simulink model "battery_pack_100s2p"  (R2025b)
settings: Solver=daessc  StartTime=0.0  StopTime=5970.0  MaxStep=5  RelTol=1e-3  AbsTol=1e-4
PostLoadFcn:
  | addpath(fullfile(fileparts(which(bdroot)),'generated'));
model workspace (MAT data in the model file):
  IpackTS = timeseries
  IpackTS.Name = 'unnamed'
  IpackTS.DataInfo = tsdata.datametadata
  IpackTS.DataInfo.Interpolation = tsdata.interpolation
  IpackTS.DataInfo.Interpolation.Fhandle : function handle (value not decoded)
  IpackTS.DataInfo.Interpolation.Name = 'linear'
  IpackTS.TimeInfo = tsdata.timemetadata
  IpackTS.TimeInfo.Length = 10
  IpackTS.TimeInfo.DuplicateTimes = 0
  IpackTS.TimeInfo.Time_ = [0; 60; 61; 2940; 2941; 3540; 3541; 5070; 5071; 5970]
  IpackTS.TimeInfo.Initialized = 1
  IpackTS.QualityInfo = tsdata.qualmetadata
  IpackTS.Data_ = [0; 0; -9; -9; 0; 0; 18; 18; 0; 0]
  ModuleBot.SOC_vecCell = [0 0.05 0.1 0.2 0.3 0.4 0.5 0.6 0.7 0.8 0.9 0.95 1]
  ModuleBot.T_vecCell = [273.15 298.15 323.15]
  ModuleBot.V0_matCell = [2.99  3  3.006; 3.34  3.35  3.356; 3.44  3.45  3.456; 3.54  3.55  3.556; 3.61  3.62  3.626; 3.67  3.68  3.686; 3.74  3.75  3.756; 3.82  3.83  3.836; 3.92  3.93  3.936; 4.01  4.02  4.026; 4.11  4.12  4.126; 4.16  4.17  4.176; 4.19  4.2  4.206]
  ModuleBot.V_rangeCell = [0 Inf]
  ModuleBot.R0_matCell = [0.0386100001983  0.0297000001525  0.0207900001068; 0.0339579673557  0.0261215133506  0.0182850593454; 0.0314679140664  0.0242060877434  0.0169442614204; 0.0294216763947  0.0226320587651  0.0158424411356; 0.0288354420652  0.0221811092809  0.0155267764967; 0.028667602662  0.0220520020477  0.0154364014334; 0.0286201487939  0.0220154990723  0.0154108493506; 0.0286099040538  0.0220076185029  0.015405332952; 0.028624710832  0.0220190083323  0.0154133058326; 0.0287228875985  0.0220945289219  0.0154661702453; 0.029248351272  0.0224987317477  0.0157491122234; 0.0300916107443  0.0231473928802  0.0162031750161; 0.0320320373038  0.0246400286952  0.0172480200867]
  ModuleBot.AHCell = 4.5
  ModuleBot.thermal_massCell = 63
  ModuleBot.AmbientResistance = 34
  ModuleBot.XminThermalResistance = 25
  ModuleBot.InterCellThermalResistance = 50
  ModuleBot.InterParallelAssemblyThermalResistance = [50 142.857142857 142.857142857 50 50 142.857142857 142.857142857 50 50 142.857142857 142.857142857 50 50 142.857142857 142.857142857 50 50 142.857142857 142.857142857 50 50 142.857142857 142.857142857 50 50 142.857142857 142.857142857 50 50 142.857142857 142.857142857 50 50 142.857142857 142.857142857 50]
  ModuleBot.InterCellRadiationArea = 0.00045
  ModuleBot.InterCellRadiationCoefficient = 4.8198179e-08
  ModuleBot.InterParallelAssemblyRadiationArea = [0.00045 0.00012 0.00012 0.00045 0.00045 0.00012 0.00012 0.00045 0.00045 0.00012 0.00012 0.00045 0.00045 0.00012 0.00012 0.00045 0.00045 0.00012 0.00012 0.00045 0.00045 0.00012 0.00012 0.00045 0.00045 0.00012 0.00012 0.00045 0.00045 0.00012 0.00012 0.00045 0.00045 0.00012 0.00012 0.00045]
  ModuleBot.InterParallelAssemblyRadiationCoefficient = 4.8198179e-08
  ModuleMid.SOC_vecCell = [0 0.05 0.1 0.2 0.3 0.4 0.5 0.6 0.7 0.8 0.9 0.95 1]
  ModuleMid.T_vecCell = [273.15 298.15 323.15]
  ModuleMid.V0_matCell = [2.99  3  3.006; 3.34  3.35  3.356; 3.44  3.45  3.456; 3.54  3.55  3.556; 3.61  3.62  3.626; 3.67  3.68  3.686; 3.74  3.75  3.756; 3.82  3.83  3.836; 3.92  3.93  3.936; 4.01  4.02  4.026; 4.11  4.12  4.126; 4.16  4.17  4.176; 4.19  4.2  4.206]
  ModuleMid.V_rangeCell = [0 Inf]
  ModuleMid.R0_matCell = [0.0386100001983  0.0297000001525  0.0207900001068; 0.0339579673557  0.0261215133506  0.0182850593454; 0.0314679140664  0.0242060877434  0.0169442614204; 0.0294216763947  0.0226320587651  0.0158424411356; 0.0288354420652  0.0221811092809  0.0155267764967; 0.028667602662  0.0220520020477  0.0154364014334; 0.0286201487939  0.0220154990723  0.0154108493506; 0.0286099040538  0.0220076185029  0.015405332952; 0.028624710832  0.0220190083323  0.0154133058326; 0.0287228875985  0.0220945289219  0.0154661702453; 0.029248351272  0.0224987317477  0.0157491122234; 0.0300916107443  0.0231473928802  0.0162031750161; 0.0320320373038  0.0246400286952  0.0172480200867]
  ModuleMid.AHCell = 4.5
  ModuleMid.thermal_massCell = 63
  ModuleMid.AmbientResistance = 34
  ModuleMid.XminThermalResistance = 25
  ModuleMid.XmaxThermalResistance = 25
  ModuleMid.InterCellThermalResistance = 50
  ModuleMid.InterParallelAssemblyThermalResistance = [50 142.857142857 142.857142857 50 50 142.857142857 142.857142857 50 50 142.857142857 142.857142857 50 50 142.857142857 142.857142857 50 50 142.857142857 142.857142857 50 50 142.857142857 142.857142857 50 50 142.857142857 142.857142857 50 50 142.857142857 142.857142857 50 50 142.857142857 142.857142857 50]
  ModuleMid.InterCellRadiationArea = 0.00045
  ModuleMid.InterCellRadiationCoefficient = 4.8198179e-08
  ModuleMid.InterParallelAssemblyRadiationArea = [0.00045 0.00012 0.00012 0.00045 0.00045 0.00012 0.00012 0.00045 0.00045 0.00012 0.00012 0.00045 0.00045 0.00012 0.00012 0.00045 0.00045 0.00012 0.00012 0.00045 0.00045 0.00012 0.00012 0.00045 0.00045 0.00012 0.00012 0.00045 0.00045 0.00012 0.00012 0.00045 0.00045 0.00012 0.00012 0.00045]
  ModuleMid.InterParallelAssemblyRadiationCoefficient = 4.8198179e-08
  ModuleTop.SOC_vecCell = [0 0.05 0.1 0.2 0.3 0.4 0.5 0.6 0.7 0.8 0.9 0.95 1]
  ModuleTop.T_vecCell = [273.15 298.15 323.15]
  ModuleTop.V0_matCell = [2.99  3  3.006; 3.34  3.35  3.356; 3.44  3.45  3.456; 3.54  3.55  3.556; 3.61  3.62  3.626; 3.67  3.68  3.686; 3.74  3.75  3.756; 3.82  3.83  3.836; 3.92  3.93  3.936; 4.01  4.02  4.026; 4.11  4.12  4.126; 4.16  4.17  4.176; 4.19  4.2  4.206]
  ModuleTop.V_rangeCell = [0 Inf]
  ModuleTop.R0_matCell = [0.0386100001983  0.0297000001525  0.0207900001068; 0.0339579673557  0.0261215133506  0.0182850593454; 0.0314679140664  0.0242060877434  0.0169442614204; 0.0294216763947  0.0226320587651  0.0158424411356; 0.0288354420652  0.0221811092809  0.0155267764967; 0.028667602662  0.0220520020477  0.0154364014334; 0.0286201487939  0.0220154990723  0.0154108493506; 0.0286099040538  0.0220076185029  0.015405332952; 0.028624710832  0.0220190083323  0.0154133058326; 0.0287228875985  0.0220945289219  0.0154661702453; 0.029248351272  0.0224987317477  0.0157491122234; 0.0300916107443  0.0231473928802  0.0162031750161; 0.0320320373038  0.0246400286952  0.0172480200867]
  ModuleTop.AHCell = 4.5
  ModuleTop.thermal_massCell = 63
  ModuleTop.AmbientResistance = 34
  ModuleTop.XmaxThermalResistance = 25
  ModuleTop.InterCellThermalResistance = 50
  ModuleTop.InterParallelAssemblyThermalResistance = [50 142.857142857 142.857142857 50 50 142.857142857 142.857142857 50 50 142.857142857 142.857142857 50 50 142.857142857 142.857142857 50 50 142.857142857 142.857142857 50 50 142.857142857 142.857142857 50 50 142.857142857 142.857142857 50 50 142.857142857 142.857142857 50 50 142.857142857 142.857142857 50]
  ModuleTop.InterCellRadiationArea = 0.00045
  ModuleTop.InterCellRadiationCoefficient = 4.8198179e-08
  ModuleTop.InterParallelAssemblyRadiationArea = [0.00045 0.00012 0.00012 0.00045 0.00045 0.00012 0.00012 0.00045 0.00045 0.00012 0.00012 0.00045 0.00045 0.00012 0.00012 0.00045 0.00045 0.00012 0.00012 0.00045 0.00045 0.00012 0.00012 0.00045 0.00045 0.00012 0.00012 0.00045 0.00045 0.00012 0.00012 0.00045 0.00045 0.00012 0.00012 0.00045]
  ModuleTop.InterParallelAssemblyRadiationCoefficient = 4.8198179e-08
  ParallelAssemblyType1.SOC_vecCell = [0 0.05 0.1 0.2 0.3 0.4 0.5 0.6 0.7 0.8 0.9 0.95 1]
  ParallelAssemblyType1.T_vecCell = [273.15 298.15 323.15]
  ParallelAssemblyType1.V0_matCell = [2.99  3  3.006; 3.34  3.35  3.356; 3.44  3.45  3.456; 3.54  3.55  3.556; 3.61  3.62  3.626; 3.67  3.68  3.686; 3.74  3.75  3.756; 3.82  3.83  3.836; 3.92  3.93  3.936; 4.01  4.02  4.026; 4.11  4.12  4.126; 4.16  4.17  4.176; 4.19  4.2  4.206]
  ParallelAssemblyType1.V_rangeCell = [0 Inf]
  ParallelAssemblyType1.R0_matCell = [0.0386100001983  0.0297000001525  0.0207900001068; 0.0339579673557  0.0261215133506  0.0182850593454; 0.0314679140664  0.0242060877434  0.0169442614204; 0.0294216763947  0.0226320587651  0.0158424411356; 0.0288354420652  0.0221811092809  0.0155267764967; 0.028667602662  0.0220520020477  0.0154364014334; 0.0286201487939  0.0220154990723  0.0154108493506; 0.0286099040538  0.0220076185029  0.015405332952; 0.028624710832  0.0220190083323  0.0154133058326; 0.0287228875985  0.0220945289219  0.0154661702453; 0.029248351272  0.0224987317477  0.0157491122234; 0.0300916107443  0.0231473928802  0.0162031750161; 0.0320320373038  0.0246400286952  0.0172480200867]
  ParallelAssemblyType1.AHCell = 4.5
  ParallelAssemblyType1.thermal_massCell = 63
  ParallelAssemblyType1.AmbientResistance = 34
  ParallelAssemblyType1.XminThermalResistance = 25
  ParallelAssemblyType1.InterCellThermalResistance = 50
  ParallelAssemblyType1.InterCellRadiationArea = 0.00045
  ParallelAssemblyType1.InterCellRadiationCoefficient = 4.8198179e-08
libraries: batt21700_mid_lib x8, fl_lib x4, nesl_utility x3, batt21700_top_lib x1, batt21700_bot_lib x1
settings Model: Creator=nhamb  LastModifiedBy=nhamb
settings SimscapeCC: SimscapeLogType=all

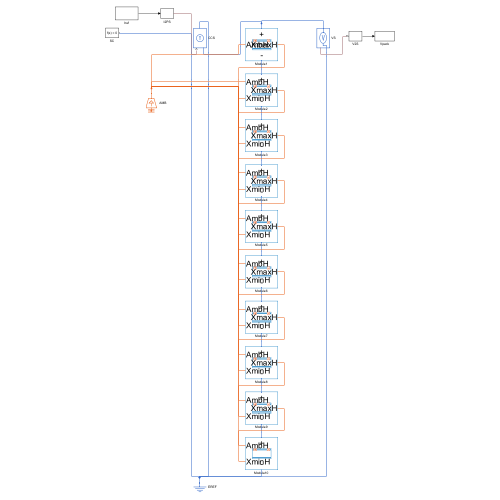
[thumbnail: Simulink's stored preview of the top-level diagram]
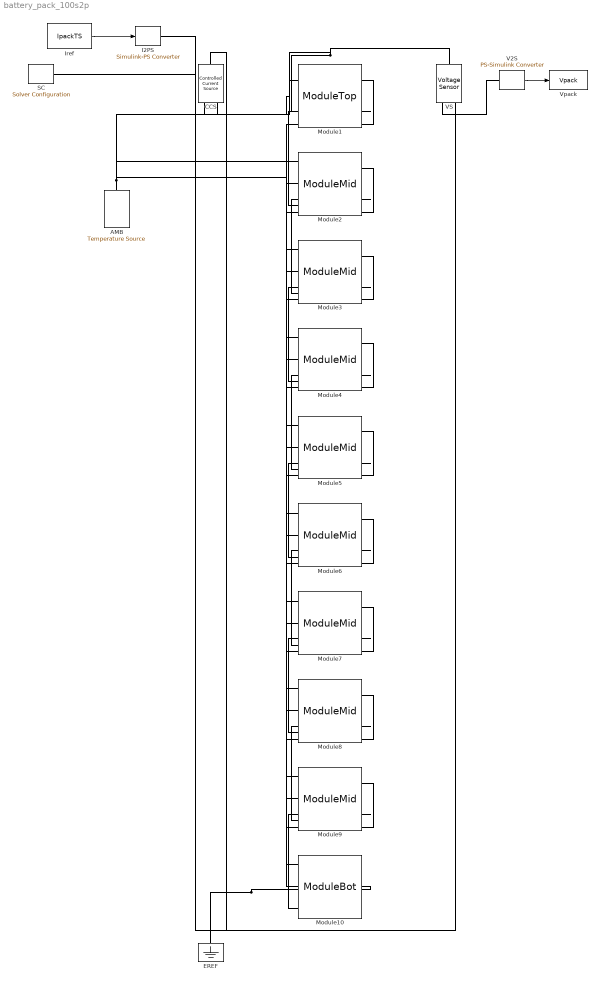
== system battery_pack_100s2p ==
  AMB : fl_lib/Thermal/Thermal Sources/Temperature Source  temperature=298.1500 K
  CCS : fl_lib/Electrical/Electrical Sources/Controlled Current Source
  EREF : fl_lib/Electrical/Electrical Elements/Electrical Reference
  I2PS : nesl_utility/Simulink-PS Converter  PhysicalDomain=network_engine_domain  SubClassName=ps_input  LeftPortType=input  RightPortType=output  PseudoPeriodic=off  Frequencies=[]  NoiseDistribution=none  NoiseParameters=[]  Unit=A  AffineConversion=off  FilteringAndDerivatives=provide  SimscapeFilterOrder=1  InputFilterTimeConstant=0.001  UdotUserProvided=0
  Iref : FromWorkspace  VariableName=IpackTS  OutputAfterFinalValue=Holding final value
  Module1 : batt21700_top_lib/ModuleTop  SOC_vecCell=ModuleTop.SOC_vecCell  T_vecCell=ModuleTop.T_vecCell K  V0_matCell=ModuleTop.V0_matCell V  V_rangeCell=ModuleTop.V_rangeCell V  R0_matCell=ModuleTop.R0_matCell Ohm  AHCell=ModuleTop.AHCell A*hr  extrapolation_optionCell=simscape.enum.extrapolation.nearest  thermal_massCell=ModuleTop.thermal_massCell J/K  AmbientResistance=[22.2034 26.9369 26.9369 34.2356 26.9369 34.2356 26.9369 34.2356 26.9369 34.2356 26.9369 34.2356 26.9369 34.2356 26.9369 34.2356 26.9369 34.2356 22.2034 26.9369] K/W  XmaxThermalResistance=ModuleTop.XmaxThermalResistance K/W  InterCellThermalResistance=ModuleTop.InterCellThermalResistance K/W  InterParallelAssemblyThermalResistance=ModuleTop.InterParallelAssemblyThermalResistance K/W  InterCellRadiationArea=ModuleTop.InterCellRadiationArea m^2  InterCellRadiationCoefficient=ModuleTop.InterCellRadiationCoefficient W/(K^4*m^2)  InterParallelAssemblyRadiationArea=ModuleTop.InterParallelAssemblyRadiationArea m^2  InterParallelAssemblyRadiationCoefficient=ModuleTop.InterParallelAssemblyRadiationCoefficient W/(K^4*m^2)  P=2  S=10  NumInterCellThermalConnections=10  NumInterParallelAssemblyThermalConnections=36  InterParallelAssemblyConnectionsMapping=[1, 1, 1, 1, 2, 2, 2, 2, 3, 3, 3, 3, 4, 4, 4, 4, 5, 5, 5, 5, 6, 6, 6, 6, 7, 7, 7, 7, 8, 8, 8, 8, 9, 9, 9, 9; 2, 2, 2, 2, 3, 3, 3, 3, 4, 4, 4, 4, 5, 5, 5, 5, 6, 6, 6, 6, 7, 7, 7, 7, 8, 8, 8, 8, 9, 9, 9, 9, 10, 10, 10, 10]  InterParallelAssemblyCellConnectionsMapping=[1, 1, 2, 2, 1, 1, 2, 2, 1, 1, 2, 2, 1, 1, 2, 2, 1, 1, 2, 2, 1, 1, 2, 2, 1, 1, 2, 2, 1, 1, 2, 2, 1, 1, 2, 2; 1, 2, 1, 2, 1, 2, 1, 2, 1, 2, 1, 2, 1, 2, 1, 2, 1, 2, 1, 2, 1, 2, 1, 2, 1, 2, 1, 2, 1, 2, 1, 2, 1, 2, 1, 2]  InterCellConnectionsMapping=[1, 1, 1, 1, 1, 1, 1, 1, 1, 1; 2, 2, 2, 2, 2, 2, 2, 2, 2, 2]  NumXmaxConnections=10  XmaxConnectionsMapping=[2, 4, 6, 8, 10, 12, 14, 16, 18, 20]  NumCellsAtXmaxBoundary=10  CellsInModelAtXmaxBoundary=[1, 1, 1, 1, 1, 1, 1, 1, 1, 1]  iCell_specify=off  iCell_priority=None  iCell=repmat(0, 20, 1) A  iCell_nominal_specify=off  iCell_nominal_value=1  iCell_nominal_unit=A  vCell_specify=off  vCell_priority=None  vCell=repmat(0, 20, 1) V  vCell_nominal_specify=off  vCell_nominal_value=1  vCell_nominal_unit=V  socCell_specify=on  socCell_priority=High  socCell=repmat(0.1500,20,1)  socCell_nominal_specify=off  socCell_nominal_value=1  socCell_nominal_unit=1  numCyclesCell_specify=off  numCyclesCell_priority=High  numCyclesCell=repmat(0, 20, 1)  numCyclesCell_nominal_specify=off  numCyclesCell_nominal_value=1  numCyclesCell_nominal_unit=1  temperatureCell_specify=on  temperatureCell_priority=High  temperatureCell=repmat(298.1500,20,1) K  temperatureCell_nominal_specify=off  temperatureCell_nominal_value=1  temperatureCell_nominal_unit=K  vParallelAssembly_specify=off  vParallelAssembly_priority=None  vParallelAssembly=repmat(0, 10, 1) V  vParallelAssembly_nominal_specify=off  vParallelAssembly_nominal_value=1  vParallelAssembly_nominal_unit=V  socParallelAssembly_specify=off  socParallelAssembly_priority=None  socParallelAssembly=repmat(1, 10, 1)  socParallelAssembly_nominal_specify=off  socParallelAssembly_nominal_value=1  socParallelAssembly_nominal_unit=1
      settings: InternalSimscapePortConfiguration="{\"Bottom\":[{\"id\":\"n\",\"label\":\"-\",\"type\":\"foundation.electrical.electrical\"}],\"Left\":[{\"id\":\"AmbH\",\"label\":\"AmbH\",\"type\":\"foundation.thermal.thermal\"}],\"Right\":[{\"id\":\"XmaxH\",\"label\":\"XmaxH\",\"type\":\"foundation.thermal.thermal\"}],\"Top\":[{\"id\":\"p\",\"label\":\"+\",\"type\":\"foundation.electrical.electrical\"}]}"
  Module10 : batt21700_bot_lib/ModuleBot  SOC_vecCell=ModuleBot.SOC_vecCell  T_vecCell=ModuleBot.T_vecCell K  V0_matCell=ModuleBot.V0_matCell V  V_rangeCell=ModuleBot.V_rangeCell V  R0_matCell=ModuleBot.R0_matCell Ohm  AHCell=ModuleBot.AHCell A*hr  extrapolation_optionCell=simscape.enum.extrapolation.nearest  thermal_massCell=ModuleBot.thermal_massCell J/K  AmbientResistance=[26.9369 22.2034 34.2356 26.9369 34.2356 26.9369 34.2356 26.9369 34.2356 26.9369 34.2356 26.9369 34.2356 26.9369 34.2356 26.9369 34.2356 26.9369 26.9369 22.2034] K/W  XminThermalResistance=ModuleBot.XminThermalResistance K/W  InterCellThermalResistance=ModuleBot.InterCellThermalResistance K/W  InterParallelAssemblyThermalResistance=ModuleBot.InterParallelAssemblyThermalResistance K/W  InterCellRadiationArea=ModuleBot.InterCellRadiationArea m^2  InterCellRadiationCoefficient=ModuleBot.InterCellRadiationCoefficient W/(K^4*m^2)  InterParallelAssemblyRadiationArea=ModuleBot.InterParallelAssemblyRadiationArea m^2  InterParallelAssemblyRadiationCoefficient=ModuleBot.InterParallelAssemblyRadiationCoefficient W/(K^4*m^2)  P=2  S=10  NumInterCellThermalConnections=10  NumInterParallelAssemblyThermalConnections=36  InterParallelAssemblyConnectionsMapping=[1, 1, 1, 1, 2, 2, 2, 2, 3, 3, 3, 3, 4, 4, 4, 4, 5, 5, 5, 5, 6, 6, 6, 6, 7, 7, 7, 7, 8, 8, 8, 8, 9, 9, 9, 9; 2, 2, 2, 2, 3, 3, 3, 3, 4, 4, 4, 4, 5, 5, 5, 5, 6, 6, 6, 6, 7, 7, 7, 7, 8, 8, 8, 8, 9, 9, 9, 9, 10, 10, 10, 10]  InterParallelAssemblyCellConnectionsMapping=[1, 1, 2, 2, 1, 1, 2, 2, 1, 1, 2, 2, 1, 1, 2, 2, 1, 1, 2, 2, 1, 1, 2, 2, 1, 1, 2, 2, 1, 1, 2, 2, 1, 1, 2, 2; 1, 2, 1, 2, 1, 2, 1, 2, 1, 2, 1, 2, 1, 2, 1, 2, 1, 2, 1, 2, 1, 2, 1, 2, 1, 2, 1, 2, 1, 2, 1, 2, 1, 2, 1, 2]  InterCellConnectionsMapping=[1, 1, 1, 1, 1, 1, 1, 1, 1, 1; 2, 2, 2, 2, 2, 2, 2, 2, 2, 2]  NumXminConnections=10  XminConnectionsMapping=[1, 3, 5, 7, 9, 11, 13, 15, 17, 19]  NumCellsAtXminBoundary=10  CellsInModelAtXminBoundary=[1, 1, 1, 1, 1, 1, 1, 1, 1, 1]  iCell_specify=off  iCell_priority=None  iCell=repmat(0, 20, 1) A  iCell_nominal_specify=off  iCell_nominal_value=1  iCell_nominal_unit=A  vCell_specify=off  vCell_priority=None  vCell=repmat(0, 20, 1) V  vCell_nominal_specify=off  vCell_nominal_value=1  vCell_nominal_unit=V  socCell_specify=on  socCell_priority=High  socCell=repmat(0.1500,20,1)  socCell_nominal_specify=off  socCell_nominal_value=1  socCell_nominal_unit=1  numCyclesCell_specify=off  numCyclesCell_priority=High  numCyclesCell=repmat(0, 20, 1)  numCyclesCell_nominal_specify=off  numCyclesCell_nominal_value=1  numCyclesCell_nominal_unit=1  temperatureCell_specify=on  temperatureCell_priority=High  temperatureCell=repmat(298.1500,20,1) K  temperatureCell_nominal_specify=off  temperatureCell_nominal_value=1  temperatureCell_nominal_unit=K  vParallelAssembly_specify=off  vParallelAssembly_priority=None  vParallelAssembly=repmat(0, 10, 1) V  vParallelAssembly_nominal_specify=off  vParallelAssembly_nominal_value=1  vParallelAssembly_nominal_unit=V  socParallelAssembly_specify=off  socParallelAssembly_priority=None  socParallelAssembly=repmat(1, 10, 1)  socParallelAssembly_nominal_specify=off  socParallelAssembly_nominal_value=1  socParallelAssembly_nominal_unit=1
      settings: InternalSimscapePortConfiguration="{\"Bottom\":[{\"id\":\"n\",\"label\":\"-\",\"type\":\"foundation.electrical.electrical\"}],\"Left\":[{\"id\":\"AmbH\",\"label\":\"AmbH\",\"type\":\"foundation.thermal.thermal\"},{\"id\":\"XminH\",\"label\":\"XminH\",\"type\":\"foundation.thermal.thermal\"}],\"Right\":[],\"Top\":[{\"id\":\"p\",\"label\":\"+\",\"type\":\"foundation.electrical.electrical\"}]}"
  Module{2..9} (8 alike) : batt21700_mid_lib/ModuleMid  SOC_vecCell=ModuleMid.SOC_vecCell  T_vecCell=ModuleMid.T_vecCell K  V0_matCell=ModuleMid.V0_matCell V  V_rangeCell=ModuleMid.V_rangeCell V  R0_matCell=ModuleMid.R0_matCell Ohm  AHCell=ModuleMid.AHCell A*hr  extrapolation_optionCell=simscape.enum.extrapolation.nearest  thermal_massCell=ModuleMid.thermal_massCell J/K  AmbientResistance=[26.9369 26.9369 34.2356 34.2356 34.2356 34.2356 34.2356 34.2356 34.2356 34.2356 34.2356 34.2356 34.2356 34.2356 34.2356 34.2356 34.2356 34.2356 26.9369 26.9369] K/W  XminThermalResistance=ModuleMid.XminThermalResistance K/W  XmaxThermalResistance=ModuleMid.XmaxThermalResistance K/W  InterCellThermalResistance=ModuleMid.InterCellThermalResistance K/W  InterParallelAssemblyThermalResistance=ModuleMid.InterParallelAssemblyThermalResistance K/W  InterCellRadiationArea=ModuleMid.InterCellRadiationArea m^2  InterCellRadiationCoefficient=ModuleMid.InterCellRadiationCoefficient W/(K^4*m^2)  InterParallelAssemblyRadiationArea=ModuleMid.InterParallelAssemblyRadiationArea m^2  InterParallelAssemblyRadiationCoefficient=ModuleMid.InterParallelAssemblyRadiationCoefficient W/(K^4*m^2)  P=2  S=10  NumInterCellThermalConnections=10  NumInterParallelAssemblyThermalConnections=36  InterParallelAssemblyConnectionsMapping=[1, 1, 1, 1, 2, 2, 2, 2, 3, 3, 3, 3, 4, 4, 4, 4, 5, 5, 5, 5, 6, 6, 6, 6, 7, 7, 7, 7, 8, 8, 8, 8, 9, 9, 9, 9; 2, 2, 2, 2, 3, 3, 3, 3, 4, 4, 4, 4, 5, 5, 5, 5, 6, 6, 6, 6, 7, 7, 7, 7, 8, 8, 8, 8, 9, 9, 9, 9, 10, 10, 10, 10]  InterParallelAssemblyCellConnectionsMapping=[1, 1, 2, 2, 1, 1, 2, 2, 1, 1, 2, 2, 1, 1, 2, 2, 1, 1, 2, 2, 1, 1, 2, 2, 1, 1, 2, 2, 1, 1, 2, 2, 1, 1, 2, 2; 1, 2, 1, 2, 1, 2, 1, 2, 1, 2, 1, 2, 1, 2, 1, 2, 1, 2, 1, 2, 1, 2, 1, 2, 1, 2, 1, 2, 1, 2, 1, 2, 1, 2, 1, 2]  InterCellConnectionsMapping=[1, 1, 1, 1, 1, 1, 1, 1, 1, 1; 2, 2, 2, 2, 2, 2, 2, 2, 2, 2]  NumXminConnections=10  XminConnectionsMapping=[1, 3, 5, 7, 9, 11, 13, 15, 17, 19]  NumCellsAtXminBoundary=10  CellsInModelAtXminBoundary=[1, 1, 1, 1, 1, 1, 1, 1, 1, 1]  NumXmaxConnections=10  XmaxConnectionsMapping=[2, 4, 6, 8, 10, 12, 14, 16, 18, 20]  NumCellsAtXmaxBoundary=10  CellsInModelAtXmaxBoundary=[1, 1, 1, 1, 1, 1, 1, 1, 1, 1]  iCell_specify=off  iCell_priority=None  iCell=repmat(0, 20, 1) A  iCell_nominal_specify=off  iCell_nominal_value=1  iCell_nominal_unit=A  vCell_specify=off  vCell_priority=None  vCell=repmat(0, 20, 1) V  vCell_nominal_specify=off  vCell_nominal_value=1  vCell_nominal_unit=V  socCell_specify=on  socCell_priority=High  socCell=repmat(0.1500,20,1)  socCell_nominal_specify=off  socCell_nominal_value=1  socCell_nominal_unit=1  numCyclesCell_specify=off  numCyclesCell_priority=High  numCyclesCell=repmat(0, 20, 1)  numCyclesCell_nominal_specify=off  numCyclesCell_nominal_value=1  numCyclesCell_nominal_unit=1  temperatureCell_specify=on  temperatureCell_priority=High  temperatureCell=repmat(298.1500,20,1) K  temperatureCell_nominal_specify=off  temperatureCell_nominal_value=1  temperatureCell_nominal_unit=K  vParallelAssembly_specify=off  vParallelAssembly_priority=None  vParallelAssembly=repmat(0, 10, 1) V  vParallelAssembly_nominal_specify=off  vParallelAssembly_nominal_value=1  vParallelAssembly_nominal_unit=V  socParallelAssembly_specify=off  socParallelAssembly_priority=None  socParallelAssembly=repmat(1, 10, 1)  socParallelAssembly_nominal_specify=off  socParallelAssembly_nominal_value=1  socParallelAssembly_nominal_unit=1
      settings: InternalSimscapePortConfiguration="{\"Bottom\":[{\"id\":\"n\",\"label\":\"-\",\"type\":\"foundation.electrical.electrical\"}],\"Left\":[{\"id\":\"AmbH\",\"label\":\"AmbH\",\"type\":\"foundation.thermal.thermal\"},{\"id\":\"XminH\",\"label\":\"XminH\",\"type\":\"foundation.thermal.thermal\"}],\"Right\":[{\"id\":\"XmaxH\",\"label\":\"XmaxH\",\"type\":\"foundation.thermal.thermal\"}],\"Top\":[{\"id\":\"p\",\"label\":\"+\",\"type\":\"foundation.electrical.electrical\"}]}"
  SC : nesl_utility/Solver Configuration  PhysicalDomain=network_engine_domain  SubClassName=solver  LeftPortType=input  RightPortType=generic  Tones=[]  Harmonics=[]  SimulateNoise=off  Profile=off  UseLocalSampling=off  EnableSwitchedLinearOptims=on  FrequencyDomain=off  UseCCode=off  RelTol=0.001  AbsTol=0.001  MinStep=1e-09  ToWorkspace=off  RevertToSquareIcSolve=off  NumHomotopyIterations=100  PhasorMode=off  PhasorModeNumHarmonics=1  ConsistencySolver=NEWTON_XTOL_AFTER_FTOL  IndexReductionMethod=DerivativeReplacement  DoDC=off  ResidualTolerance=1e-09  ConsistencyTolSource=GLOBAL  ConsistencyAbsTol=0.001  ConsistencyRelTol=0.001  ConsistencyTolFactor=0.001  UseLocalSolver=off  LocalSolverChoice=NE_BACKWARD_EULER_ADVANCER  ResolveIndetEquations=on  FunctionEvalNumThread=1  LocalSolverSampleTime=0.001  DoFixedCost=off  MaxNonlinIter=3  MaxModeIter=2  ComputeImpulses=off  ImpulseIterations=2  LinearAlgebra=auto  LinearAlgebraNumThread=0  EquationFormulation=NE_TIME_EF  DelaysMemoryBudget=1024  AutomaticFiltering=on  FilteringTimeConstant=0.001  PartitionStorageMethod=AS_NEEDED  PartitionMemoryBudget=1024  PartitionMethod=ROBUST  MultibodyUseLocalSolver=off  MultibodyLocalSolverChoice=ODE1  MultibodyLocalSolverSampleTime=0.001
  V2S : nesl_utility/PS-Simulink Converter  PhysicalDomain=network_engine_domain  SubClassName=ps_output  LeftPortType=input  RightPortType=output  PseudoPeriodic=off  Frequencies=[]  VectorFormat=inherit  Unit=V  AffineConversion=off
  VS : fl_lib/Electrical/Electrical Sensors/Voltage Sensor
  Vpack : ToWorkspace  VariableName=Vpack  SaveFormat=Structure With Time  SampleTime=-1
  wires:
  Iref/1 -> I2PS/1
  V2S/1 -> Vpack/1
  connections:
  Module1/LConn2 -- CCS/RConn2 -- VS/LConn1
  Module1/RConn2 -- Module2/LConn3
  Module2/RConn2 -- Module3/LConn3
  Module3/RConn2 -- Module4/LConn3
  Module4/RConn2 -- Module5/LConn3
  Module5/RConn2 -- Module6/LConn3
  Module6/RConn2 -- Module7/LConn3
  Module7/RConn2 -- Module8/LConn3
  Module8/RConn2 -- Module9/LConn3
  Module9/RConn2 -- Module10/LConn3
  Module10/RConn1 -- CCS/LConn1 -- VS/RConn2 -- EREF/LConn1 -- SC/RConn1
  Module1/RConn1 -- Module2/LConn2
  Module2/RConn1 -- Module3/LConn2
  Module3/RConn1 -- Module4/LConn2
  Module4/RConn1 -- Module5/LConn2
  Module5/RConn1 -- Module6/LConn2
  Module6/RConn1 -- Module7/LConn2
  Module7/RConn1 -- Module8/LConn2
  Module8/RConn1 -- Module9/LConn2
  Module9/RConn1 -- Module10/LConn2
  Module1/LConn1 -- AMB/LConn1 -- Module2/LConn1 -- Module3/LConn1 -- Module4/LConn1 -- Module5/LConn1 -- Module6/LConn1 -- Module7/LConn1 -- Module8/LConn1 -- Module9/LConn1 -- Module10/LConn1
  I2PS/RConn1 -- CCS/RConn1
  VS/RConn1 -- V2S/LConn1
